simulink model "sorosimulink"  (R2024b)
settings: Solver=ode15s  StartTime=0.0  StopTime=100.0  RelTol=1e-3
values from neighbouring files (symbols this model uses):
  x0 = [zeros(T1.ndof, 1); zeros(T1.ndof, 1)]    [simulation.m]
settings Model: Creator=danie  LastModifiedBy=d.caradonna
settings RTWCC: GPUComputeCapability=3.5

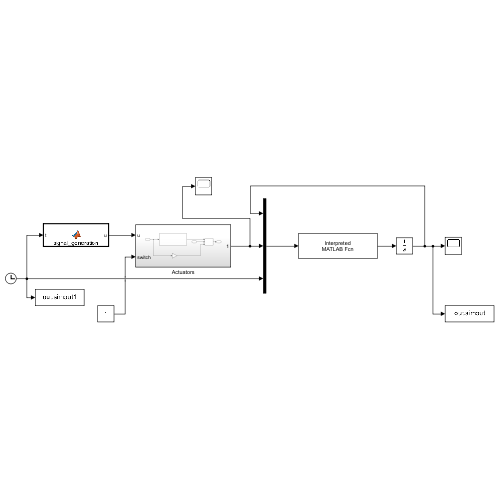
[thumbnail: Simulink's stored preview of the top-level diagram]
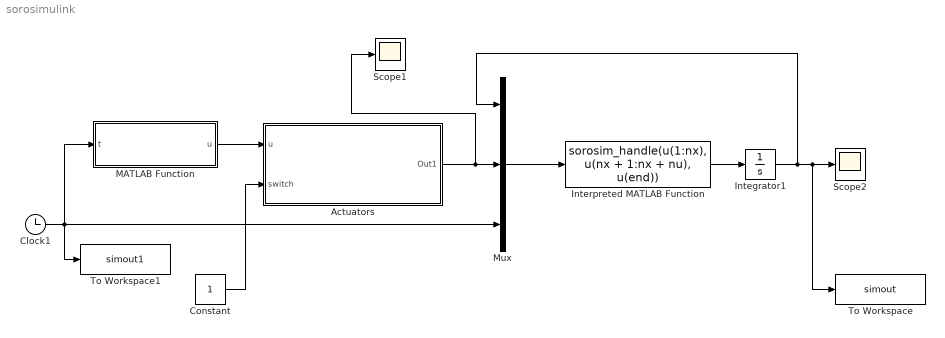
== system sorosimulink ==
  Actuators : Subsystem
  Clock1 : Clock
  Constant : Constant
  Integrator1 : Integrator  InitialCondition=x0
  Interpreted MATLAB Function : MATLABFcn  MATLABFcn=sorosim_handle(u(1:nx), u(nx + 1:nx + nu), u(end))
  MATLAB Function : MATLAB Function  TreatAsAtomicUnit=on
  Mux : Mux  Inputs=3
  Scope1 : Scope
  Scope2 : Scope
  To Workspace : ToWorkspace  VariableName=simout  SaveFormat=Timeseries  SampleTime=-1
  To Workspace1 : ToWorkspace  VariableName=simout1  SaveFormat=Timeseries  SampleTime=-1
  wires:
  Integrator1/1 -> To Workspace/1, Scope2/1, Mux/1
  Clock1/1 -> To Workspace1/1, Mux/3, MATLAB Function/1(t)
  Interpreted MATLAB Function/1 -> Integrator1/1
  Mux/1 -> Interpreted MATLAB Function/1
  MATLAB Function/1(u) -> Actuators/1(u)
  Actuators/1(Out1) -> Scope1/1, Mux/2
  Constant/1 -> Actuators/2(switch)

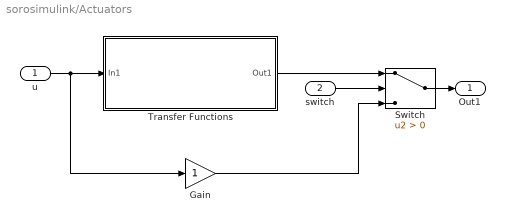
== system sorosimulink/Actuators ==
  u : Inport
  switch : Inport  Port=2
  Gain : Gain
  Switch : Switch  Criteria=u2 > Threshold  SaturateOnIntegerOverflow=off  InputSameDT=off
  Transfer Functions : Subsystem
  Out1 : Outport
  wires:
  Switch/1 -> Out1/1
  switch/1 -> Switch/2
  Gain/1 -> Switch/3
  u/1 -> Gain/1, Transfer Functions/1(In1)
  Transfer Functions/1(Out1) -> Switch/1

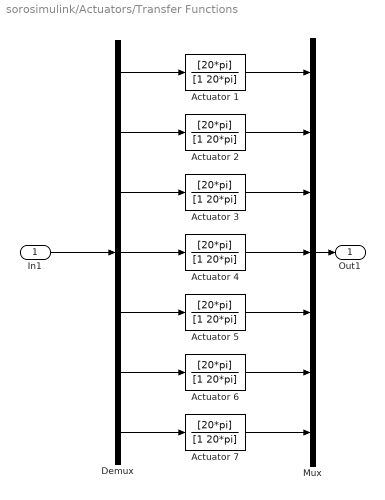
== system sorosimulink/Actuators/Transfer Functions ==
  In1 : Inport
  Actuator {1..7} (7 alike) : TransferFcn  Numerator=[20*pi]  Denominator=[1 20*pi]
  Demux : Demux  Outputs=7
  Mux : Mux  Inputs=7
  Out1 : Outport
  wires:
  Demux/4 -> Actuator 4/1
  Actuator 2/1 -> Mux/2
  Demux/2 -> Actuator 2/1
  Actuator 4/1 -> Mux/4
  Actuator 3/1 -> Mux/3
  Actuator 6/1 -> Mux/6
  Actuator 7/1 -> Mux/7
  Demux/1 -> Actuator 1/1
  Actuator 1/1 -> Mux/1
  Demux/3 -> Actuator 3/1
  Demux/5 -> Actuator 5/1
  Actuator 5/1 -> Mux/5
  Demux/7 -> Actuator 7/1
  Demux/6 -> Actuator 6/1
  In1/1 -> Demux/1
  Mux/1 -> Out1/1

== matlab function sorosimulink/MATLAB Function ==
  data: t input; u output
function u = signal_generation(t) 
    gain = blkdiag(2.5e+2*eye(3), 2.5e+3*eye(4));
    u = gain*chirp(t, 7, 1, 1e+0);
end
